simulink model "Two_mass_stifness_system_modal_controller_observer"  (R2018b)
settings: Solver=ode3  StartTime=0.0  StopTime=2  FixedStep=1e-5  RelTol=1e-3  EnableMultiTasking=on
values from neighbouring files (symbols this model uses):
  c = GJp/l    (= 0.0104)    [params.m]
  ce = (Un - In*R)/wn    (= 0.301701587302)    [params.m]
  cm = Mn/In    (= 0.212068965517)    [params.m]
  Jadd = Jm/10    (= 5.9e-06)    [params.m]
  Jm = 0.59*10^(-4)    (= 5.9e-05)    [params.m]
  K = place(A,B,p)    [script.m]
  L = 130*10^(-3)    (= 0.13)    [params.m]    (also in script.m = l')
  R = 25.8    [params.m]
undefined symbols (not defined in the file or in its folder): A, B, C
settings Model: Creator=user  LastModifiedBy=user
settings DataIOCC: SaveFormat=Array  OutputSaveName=x1
settings OptimizationCC: LifeSpan=inf
settings DebuggingCC: UnderspecifiedInitializationDetection=Classic  MergeDetectMultiDrivingBlocksExec=none  SolverPrmCheckMsg=warning  SFUnexpectedBacktrackingDiag=warning  SFNoUnconditionalDefaultTransitionDiag=warning  SFExecutionAtInitializationDiag=none
settings HardwareCC: ProdBitPerPointer=32  ProdBitPerSizeT=32  ProdBitPerPtrDiffT=32  ProdLargestAtomicFloat=None  ProdIntDivRoundTo=Undefined  ProdEndianess=Unspecified  ProdWordSize=32  ProdHWDeviceType=32-bit Generic
settings ModelReferenceCC: PropagateSignalLabelsOutOfModel=off
settings SFSimCC: SimUseLocalCustomCode=off
settings RTWCC: RTWUseLocalCustomCode=off
settings CodeAppCC: StateflowObjectComments=on
settings GRTTargetCC: TargetLangStandard=C89/C90 (ANSI)  GeneratePreprocessorConditionals=Disable all
settings ConfigComp: CovMetricSettings=dw  CovHtmlReporting=on  CovSaveCumulativeToWorkspaceVar=on  CovSaveSingleToWorkspaceVar=on  CovExternalEMLEnable=off

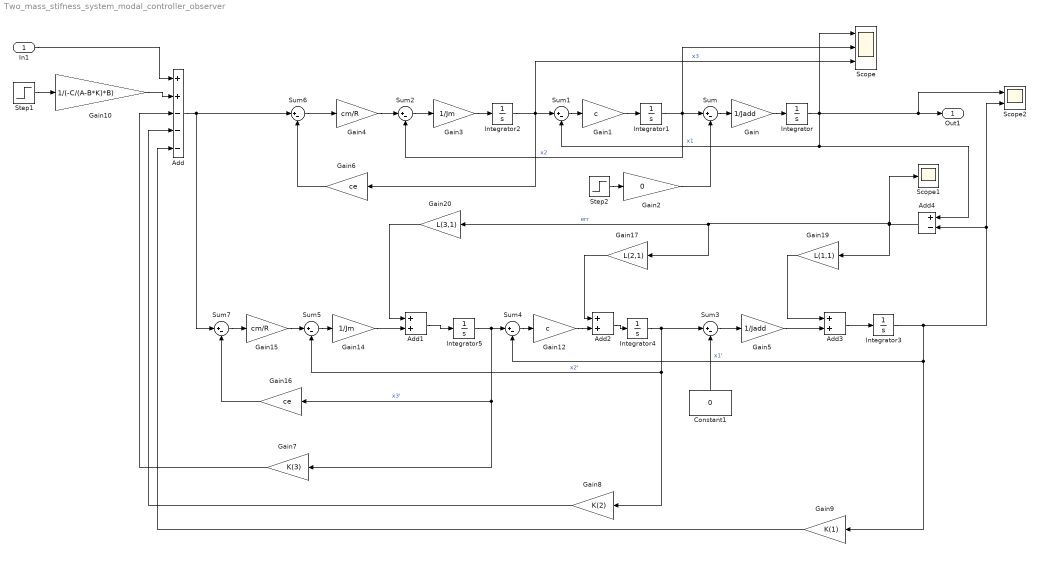
== system Two_mass_stifness_system_modal_controller_observer ==
  In1 : Inport
  Add : Sum  Inputs=++---
  Add1 : Sum
  Add2 : Sum
  Add3 : Sum
  Add4 : Sum  Inputs=+-
  Constant1 : Constant  Value=0
  Gain : Gain  Gain=1/Jadd
  Gain1 : Gain  Gain=c
  Gain10 : Gain  Gain=1/(-C/(A-B*K)*B)
  Gain12 : Gain  Gain=c
  Gain14 : Gain  Gain=1/Jm
  Gain15 : Gain  Gain=cm/R
  Gain16 : Gain  Gain=ce
  Gain17 : Gain  Gain=L(2,1)
  Gain19 : Gain  Gain=L(1,1)
  Gain2 : Gain  Gain=0
  Gain20 : Gain  Gain=L(3,1)
  Gain3 : Gain  Gain=1/Jm
  Gain4 : Gain  Gain=cm/R
  Gain5 : Gain  Gain=1/Jadd
  Gain6 : Gain  Gain=ce
  Gain7 : Gain  Gain=K(3)
  Gain8 : Gain  Gain=K(2)
  Gain9 : Gain  Gain=K(1)
  Integrator{,1..2,4..5} (5 alike) : Integrator
  Integrator3 : Integrator  InitialCondition=20
  Scope : Scope  NumInputPorts=3
  Scope1 : Scope
  Scope2 : Scope  NumInputPorts=2
  Step1 : Step  Time=0  After=10  SampleTime=0
  Step2 : Step  SampleTime=0
  Sum{,1..7} (8 alike) : Sum  Inputs=|+-
  Out1 : Outport
  wires:
  Sum/1 -> Gain/1
  Gain/1 -> Integrator/1
  Gain1/1 -> Integrator1/1
  Integrator1/1 -> Sum2/2, Scope/2, Sum/1  "x2"
  Sum1/1 -> Gain1/1
  Integrator/1 -> Add4/1, Sum1/2, Scope/1, Scope2/1, Out1/1  "x1"
  Gain3/1 -> Integrator2/1
  Integrator2/1 -> Gain6/1, Scope/3, Sum1/1  "x3"
  Sum2/1 -> Gain3/1
  Gain4/1 -> Sum2/1
  Add/1 -> Sum6/1, Sum7/1
  In1/1 -> Add/1
  Gain10/1 -> Add/2
  Gain7/1 -> Add/3
  Gain8/1 -> Add/4
  Gain9/1 -> Add/5
  Sum3/1 -> Gain5/1
  Integrator4/1 -> Sum5/2, Gain8/1, Sum3/1  "x2'"
  Sum4/1 -> Gain12/1
  Integrator3/1 -> Gain9/1, Sum4/2, Scope2/2, Add4/2  "x1'"
  Integrator5/1 -> Gain7/1, Gain16/1, Sum4/1  "x3'"
  Sum5/1 -> Gain14/1
  Gain15/1 -> Sum5/1
  Gain14/1 -> Add1/2
  Add1/1 -> Integrator5/1
  Gain12/1 -> Add2/2
  Add2/1 -> Integrator4/1
  Gain5/1 -> Add3/2
  Add3/1 -> Integrator3/1
  Gain20/1 -> Add1/1
  Gain17/1 -> Add2/1
  Gain19/1 -> Add3/1
  Add4/1 -> Scope1/1, Gain17/1, Gain20/1, Gain19/1  "err"
  Sum6/1 -> Gain4/1
  Gain6/1 -> Sum6/2
  Sum7/1 -> Gain15/1
  Gain16/1 -> Sum7/2
  Constant1/1 -> Sum3/2
  Step2/1 -> Gain2/1
  Gain2/1 -> Sum/2
  Step1/1 -> Gain10/1
